simulink model "LCC_TorqueControl_MPC"  (R2023b)
settings: Solver=FixedStepDiscrete  StartTime=0.0  StopTime=10.0  FixedStep=.05  RelTol=1e-3
libraries: simulink_extras x1
settings Model: Creator=balls  LastModifiedBy=scb548
settings RTWCC: Description=Generate an RTMaps component embedding the model  SystemTargetFile=rtmaps.tlc  TemplateMakefile=rtmaps_default_tmf  RetainRTWFile=on  TargetLang=C++
settings STFCustomTargetCC: TargetLangStandard=C++11 (ISO)  ModelReferenceCompliant=off  CombineOutputUpdateFcns=on  SystemTargetFile=rtmaps.tlc
settings GRTTargetCC: TargetLangStandard=C++11 (ISO)  ModelReferenceCompliant=off  ParMdlRefBuildCompliant=off  CompOptLevelCompliant=off  ConcurrentExecutionCompliant=off  MatFileLogging=off  CPPClassGenCompliant=off  UseToolchainInfoCompliant=off

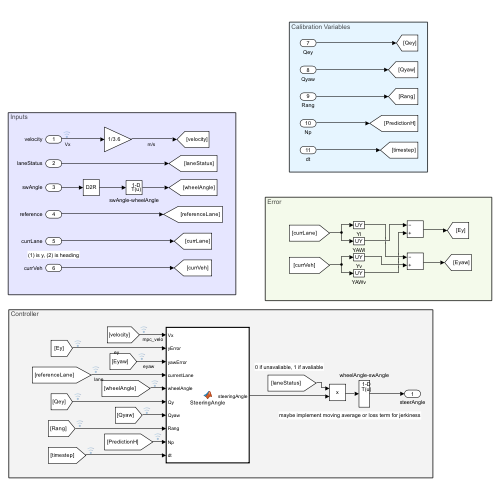
[thumbnail: Simulink's stored preview of the top-level diagram]
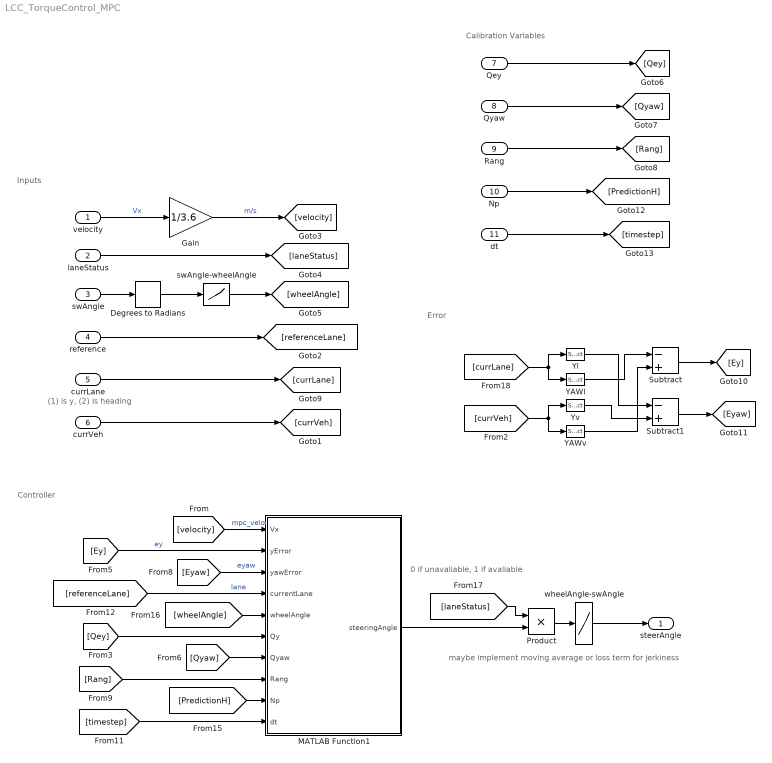
== system LCC_TorqueControl_MPC ==
  note: Error
  note: Controller
  note: 0 if unavaliable, 1 if avaliable
  note: (1) is y, (2) is heading
  note: Inputs
  note: maybe implement moving average or loss term for jerkiness
  note: Calibration Variables
  velocity : Inport
  laneStatus : Inport  Port=2
  swAngle : Inport  Port=3
  reference : Inport  Port=4  PortDimensions=[2, 11]
  currLane : Inport  Port=5
  currVeh : Inport  Port=6
  Qey : Inport  Port=7
  Qyaw : Inport  Port=8
  Rang : Inport  Port=9
  Np : Inport  Port=10
  dt : Inport  Port=11
  Degrees to Radians : simulink_extras/Transformations/Degrees to Radians
  Gain : Gain  Gain=1/3.6
  MATLAB Function1 : MATLAB Function  TreatAsAtomicUnit=on
  Product : Product
  Subtract : Sum  Inputs=-+
  Subtract1 : Sum  Inputs=-+
  YAWl : Selector  InputPortWidth=2  IndexOptions=Index vector (dialog)  Indices=2  OutputSizes=1
  YAWv : Selector  InputPortWidth=2  IndexOptions=Index vector (dialog)  Indices=2  OutputSizes=1
  Yl : Selector  InputPortWidth=2  IndexOptions=Index vector (dialog)  Indices=1  OutputSizes=1
  Yv : Selector  InputPortWidth=2  IndexOptions=Index vector (dialog)  Indices=1  OutputSizes=1
  swAngle-wheelAngle : Lookup_n-D  NumberOfTableDimensions=1  BreakpointsForDimension1=[-0.636900008;-0.589100003;-0.539099991;-0.490500003;-0.44659999;-0.404900014;-0.361499995;-0.317299992;-0.27610001;-0.237499997;-0.197899997;-0.156399995;-0.1162;-0.078699999;-0.041099999;-0.001;0.001;0.041200001;0.079099998;0.116499998;0.156399995;0.197999999;0.237900004;0.276499987;0.317400008;0.361499995;0.405299991;0.447100013;0.490700006;0.539099991;0.589399993;0.637499988]  Table=[-10.89089966;-10.16600037;-9.441100121;-8.716199875;-7.991300106;-7.26639986;-6.541500092;-5.816599846;-5.091700077;-4.366799831;-3.641900063;-2.917000055;-2.192100048;-1.467200041;-0.742299974;-0.0175;0.0175;0.742299974;1.467200041;2.192100048;2.917000055;3.641900063;4.366799831;5.091700077;5.816599846;6.541500092;7.26639986;7.991300106;8.716199875;9.441100121;10.16600037;10.89089966]  InternalRulePriority=Speed  RndMeth=Simplest
  wheelAngle-swAngle : Lookup_n-D  NumberOfTableDimensions=1  BreakpointsForDimension1=[-10.89089966;-10.16600037;-9.441100121;-8.716199875;-7.991300106;-7.26639986;-6.541500092;-5.816599846;-5.091700077;-4.366799831;-3.641900063;-2.917000055;-2.192100048;-1.467200041;-0.742299974;-0.0175;0.0175;0.742299974;1.467200041;2.192100048;2.917000055;3.641900063;4.366799831;5.091700077;5.816599846;6.541500092;7.26639986;7.991300106;8.716199875;9.441100121;10.16600037;10.89089966]  Table=[-0.636900008;-0.589100003;-0.539099991;-0.490500003;-0.44659999;-0.404900014;-0.361499995;-0.317299992;-0.27610001;-0.237499997;-0.197899997;-0.156399995;-0.1162;-0.078699999;-0.041099999;-0.001;0.001;0.041200001;0.079099998;0.116499998;0.156399995;0.197999999;0.237900004;0.276499987;0.317400008;0.361499995;0.405299991;0.447100013;0.490700006;0.539099991;0.589399993;0.637499988]  InternalRulePriority=Speed  RndMeth=Simplest
  steerAngle : Outport
  wires:
  Qey/1 -> [Qey]
  Qyaw/1 -> [Qyaw]
  Rang/1 -> [Rang]
  velocity/1 -> Gain/1  "Vx"
  laneStatus/1 -> [laneStatus]
  swAngle/1 -> Degrees to Radians/1
  Gain/1 -> [velocity]  "m/s"
  Degrees to Radians/1 -> swAngle-wheelAngle/1
  swAngle-wheelAngle/1 -> [wheelAngle]
  [laneStatus] -> Product/1
  Product/1 -> wheelAngle-swAngle/1
  currVeh/1 -> [currVeh]
  [currLane] -> YAWl/1, Yl/1
  [currVeh] -> Yv/1, YAWv/1
  YAWv/1 -> Subtract/2
  YAWl/1 -> Subtract/1
  Yl/1 -> Subtract1/1
  Yv/1 -> Subtract1/2
  Subtract/1 -> [Ey]
  Subtract1/1 -> [Eyaw]
  MATLAB Function1/1(steeringAngle) -> Product/2
  [velocity] -> MATLAB Function1/1(Vx)  "mpc_velo"
  [Qey] -> MATLAB Function1/6(Qy)
  [Ey] -> MATLAB Function1/2(yError)  "ey"
  [Qyaw] -> MATLAB Function1/7(Qyaw)
  [Eyaw] -> MATLAB Function1/3(yawError)  "eyaw"
  [Rang] -> MATLAB Function1/8(Rang)
  [referenceLane] -> MATLAB Function1/4(currentLane)  "lane"
  Np/1 -> [PredictionH]
  [PredictionH] -> MATLAB Function1/9(Np)
  [timestep] -> MATLAB Function1/10(dt)
  dt/1 -> [timestep]
  [wheelAngle] -> MATLAB Function1/5(wheelAngle)
  wheelAngle-swAngle/1 -> steerAngle/1
  currLane/1 -> [currLane]
  reference/1 -> [referenceLane]

== matlab function LCC_TorqueControl_MPC/MATLAB Function1 ==
  data: Vx input; steeringAngle output; yError input; yawError input; currentLane input; wheelAngle input; Qy input; Qyaw input; Rang input; Np input; dt input
function steeringAngle = SteeringAngle(Vx, yError, yawError, currentLane, wheelAngle, Qy, Qyaw, Rang, Np, dt)
    
    % Reference trajectory: Np steps of [yaw, lateral_y]
    refTrajectory = currentLane;

    if Vx == 0
        Vx = .01;
    end
    
    % Weight matrices
    Q = diag([Qy, Qyaw]);  % Higher weight on yaw and y errors
    R = Rang;            % Penalize steering angle magnitude
    S = Rang/2;             % Penalize steering angle rate
    
    % Vehicle parameters (Slide 42)
    m = 2721.6;
    Jz = 2624;
    lf = 1.5;
    lr = 1.5;
    Cf = 12000;
    Cr = 20000;
    
    % Continuous model (Slide 42)
    A = [-(Cf+Cr)/(m*Vx), -Vx - (Cf*lf - Cr*lr)/(m*Vx), 0, 0;
         -(Cf*lf - Cr*lr)/(Jz*Vx), -(Cf*lf^2 + Cr*lr^2)/(Jz*Vx), 0, 0;
         0, 1, 0, 0;
         1, 0, Vx, 0];
    B = [Cf/m; (Cf*lf)/Jz; 0; 0];
    C = [0 0 1 0; 0 0 0 1]; % Extract yaw and lateral position
    
    % Discretize
    Ad = eye(4) + A * dt;
    Bd = B * dt;
    
    % Initial state
    x0 = [0; 0; yawError; yError];

    persistent u0
    if isempty(u0)
        u0 = wheelAngle*ones(Np, 1);
    end
    
    % Preallocate F and G
    F = [];
    G = [];

    for i = 1:Np
        Ai = Ad^i;
        F = [F; C * Ai];
        
        Gi = zeros(2, Np);
        for j = 1:i
            Gi(:, j) = C * Ad^(i-j) * Bd;
        end
        G = [G; Gi];
    end
    
    % Construct reference vector
    yref = reshape(refTrajectory', [], 1); % [yaw1; y1; yaw2; y2; ...]
    
    % Construct weight matrices
    Qblk = kron(eye(Np), Q);
    Rblk = kron(eye(Np), R);
    Sblk = kron(eye(Np-1), S);
    
    % Construct delta rate penalty matrix T
    T = zeros(Np - 1, Np);
    for i = 1:Np - 1
        T(i, i) = -1;
        T(i, i + 1) = 1;
    end
    
    % Cost matrices
    H = G' * Qblk * G + Rblk + T' * Sblk * T;
    f = G' * Qblk * (F * x0 - yref);
    
    % Solve with quadprog
    delta = quadprog(2*H, 2*f, [], [], [], [], [], [], u0, optimoptions('quadprog','Algorithm','active-set'));

    steeringAngle = delta(1);

    u0 = delta;

end
